simulink model "Ornek3_4"  (R2021b)
settings: Solver=VariableStepAuto  StartTime=0.0  StopTime=9  RelTol=1e-3
undefined symbols (not defined in the file or in its folder): fdesignblkfcn, gcbh
libraries: dsparch4 x1, dspsigops x1
settings Model: Creator=MONSTER  LastModifiedBy=MONSTER

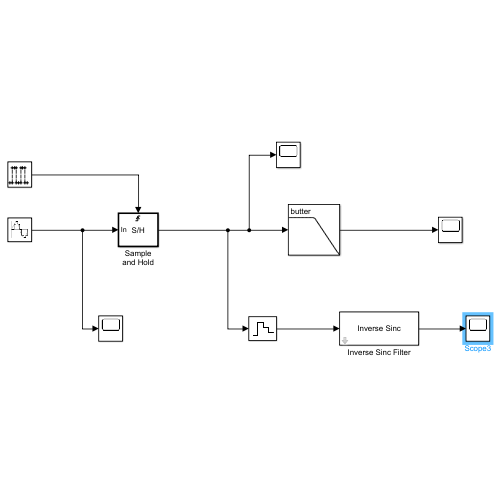
[thumbnail: Simulink's stored preview of the top-level diagram]
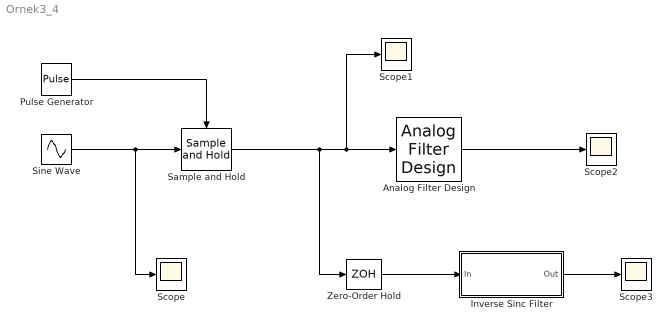
== system Ornek3_4 ==
  Analog Filter Design : dsparch4/Analog Filter Design  method=Butterworth  filttype=Lowpass  N=8  Wlo=30  Whi=80  Rp=2  Rs=40
  Inverse Sinc Filter : Subsystem  DialogController=fdesignblkfcn  InitFcn=fdesignblkfcn(gcbh, {'InitFcn'});  mask(Inverse Sinc Filter){}
      mask help: Design an inverse sinc filter
      settings: CopyFcn=fdesignblkfcn(gcbh, {'CopyFcn'});
      mask Help: helpview(mapfilelocation('dsp'), 'dspinversesincfilter');
      mask Display: disp('Inverse Sinc');
  Pulse Generator : DiscretePulseGenerator  Period=9  PulseWidth=7  SampleTime=0.001
  Sample and Hold : dspsigops/Sample and Hold  trig=Rising edge  initCond=0  latchinput=off
  Scope{,1..3} (4 alike) : Scope
  Sine Wave : Sin  Frequency=4  SampleTime=0.001
  Zero-Order Hold : ZeroOrderHold  SampleTime=-1
  wires:
  Pulse Generator/1 -> Sample and Hold/Trigger
  Sine Wave/1 -> Scope/1, Sample and Hold/1
  Sample and Hold/1 -> Scope1/1, Analog Filter Design/1, Zero-Order Hold/1
  Analog Filter Design/1 -> Scope2/1
  Zero-Order Hold/1 -> Inverse Sinc Filter/1(In)
  Inverse Sinc Filter/1(Out) -> Scope3/1

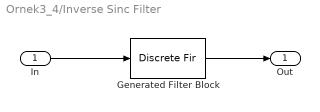
== system Ornek3_4/Inverse Sinc Filter ==
  In : Inport
  Generated Filter Block : DiscreteFir  Tag=BlockMethodSubSystem  Coefficients=[-0.0026843274692852663 -0.002346162151096788 0.0073965993169508026 0.018442797618651186 0.012351106329410911 -0.0067934613704367722 -0.0093225132104399755 0.010137634289690594 0.014452636598032568 -0.01096659610710831 -0.020288876931548214 0.012277085521236011 0.029020142443779536 -0.013203596820367916 -0.042093940662690496 0.013627754834690312 0.064277570694568714 -0.012757715101713234 -0.11270171800644833 0.0051188971746040065 0.32344134739197722 0.50160314889955848 0.32344134739197722 0.0051188971746040065 -0.11270171800644833 -0.012757715101713234 0.064277570694568714 0.013627754834690312 -0.042093940662690496 -0.013203596820367916 0.029020142443779536 0.012277085521236011 -0.020288876931548214 -0.01096659610710831 0.014452636598032568 0.010137634289690594 -0.0093225132104399755 -0.0067934613704367722 0.012351106329410911 0.018442797618651186 0.0073965993169508026 -0.002346162151096788 -0.0026843274692852663]  InputProcessing=Columns as channels (frame based)
  Out : Outport  VectorParamsAs1DForOutWhenUnconnected=off
  wires:
  Generated Filter Block/1 -> Out/1
  In/1 -> Generated Filter Block/1
